simulink model "adaptiveFinal"  (R2014b)
settings: Solver=ode45  StartTime=0.0  StopTime=50.0  RelTol=1e-3
libraries: simulink x2
settings Model: Creator=highamj  LastModifiedBy=highamj

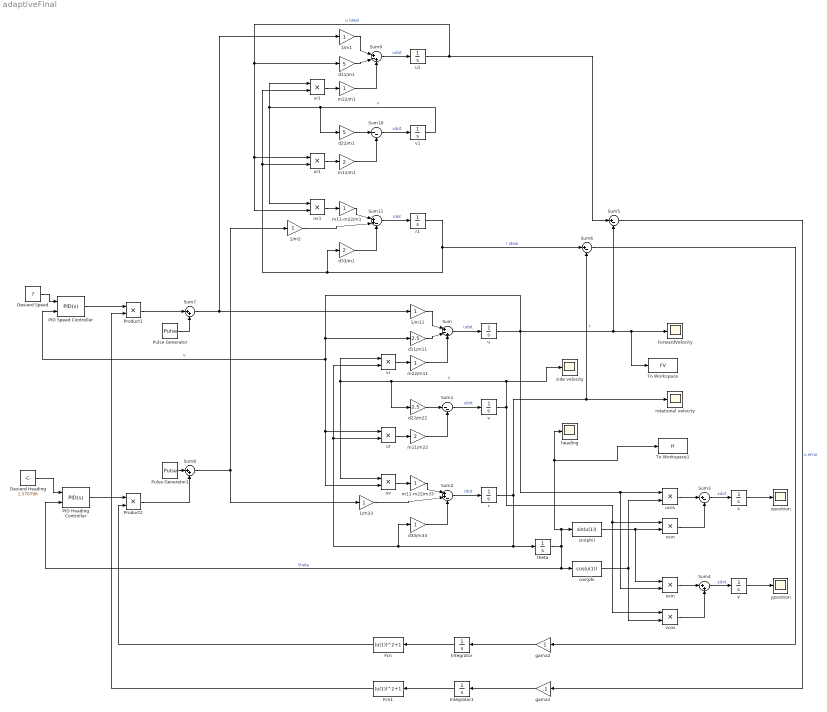
== system adaptiveFinal ==
  1/m{1..2,11,33} (4 alike) : Gain
  Desierd Heading : Constant  Value=1.570796
  Desierd Speed : Constant  Value=7
  Fcn : Fcn  Expr=(u(1))^2+1
  Fcn1 : Fcn  Expr=(u(1))^2+1
  ForwardVelocity : Scope
      settings: YMin=-2.92e+11  YMax=-2.86e+11  SaveName=ScopeData3
  Integrator : Integrator
  Integrator1 : Integrator
  PID Heading Controller : simulink/Continuous/PID Controller (2DOF)  Controller=PID  TimeDomain=Continuous-time  SampleTime=-1  IntegratorMethod=Forward Euler  FilterMethod=Forward Euler  Form=Parallel  P=5.96375779922345  I=0.127939709833734  D=1.41156755886535  N=5.23154506794489  b=1  c=1  InitialConditionSource=internal  InitialConditionForIntegrator=0  InitialConditionForFilter=0  ExternalReset=none  LimitOutput=off  UpperSaturationLimit=inf  LowerSaturationLimit=-inf  LinearizeAsGain=on  AntiWindupMode=none  Kb=1  TrackingMode=off  Kt=1  PParamMin=[]  PParamMax=[]  IParamMin=[]  IParamMax=[]  DParamMin=[]  DParamMax=[]  NParamMin=[]  NParamMax=[]  bParamMin=[]  bParamMax=[]  cParamMin=[]  cParamMax=[]  KbParamMin=[]  KbParamMax=[]  KtParamMin=[]  KtParamMax=[]  POutMin=[]  POutMax=[]  IOutMin=[]  IOutMax=[]  DOutMin=[]  DOutMax=[]  NOutMin=[]  NOutMax=[]  bOutMin=[]  bOutMax=[]  cOutMin=[]  cOutMax=[]  KbOutMin=[]  KbOutMax=[]  KtOutMin=[]  KtOutMax=[]  IntegratorOutMin=[]  IntegratorOutMax=[]  FilterOutMin=[]  FilterOutMax=[]  SumOutMin=[]  SumOutMax=[]  Sum1OutMin=[]  Sum1OutMax=[]  Sum2OutMin=[]  Sum2OutMax=[]  Sum3OutMin=[]  Sum3OutMax=[]  SumI1OutMin=[]  SumI1OutMax=[]  SumI2OutMin=[]  SumI2OutMax=[]  SumI3OutMin=[]  SumI3OutMax=[]  SumDOutMin=[]  SumDOutMax=[]  SaturationOutMin=[]  SaturationOutMax=[]  IntegratorContinuousStateAttributes=''  IntegratorStateMustResolveToSignalObject=off  IntegratorRTWStateStorageClass=Auto  FilterContinuousStateAttributes=''  FilterStateMustResolveToSignalObject=off  FilterRTWStateStorageClass=Auto  DifferentiatorICPrevScaledInput=0  DifferentiatorOutMin=[]  DifferentiatorOutMax=[]  UseFilter=on
  PID Speed Controller : simulink/Continuous/PID Controller (2DOF)  Controller=PID  TimeDomain=Continuous-time  SampleTime=-1  IntegratorMethod=Forward Euler  FilterMethod=Forward Euler  Form=Parallel  P=0  I=4.52260515354749  D=0  N=100  b=1  c=1  InitialConditionSource=internal  InitialConditionForIntegrator=0  InitialConditionForFilter=0  ExternalReset=none  LimitOutput=off  UpperSaturationLimit=inf  LowerSaturationLimit=-inf  LinearizeAsGain=on  AntiWindupMode=none  Kb=1  TrackingMode=off  Kt=1  PParamMin=[]  PParamMax=[]  IParamMin=[]  IParamMax=[]  DParamMin=[]  DParamMax=[]  NParamMin=[]  NParamMax=[]  bParamMin=[]  bParamMax=[]  cParamMin=[]  cParamMax=[]  KbParamMin=[]  KbParamMax=[]  KtParamMin=[]  KtParamMax=[]  POutMin=[]  POutMax=[]  IOutMin=[]  IOutMax=[]  DOutMin=[]  DOutMax=[]  NOutMin=[]  NOutMax=[]  bOutMin=[]  bOutMax=[]  cOutMin=[]  cOutMax=[]  KbOutMin=[]  KbOutMax=[]  KtOutMin=[]  KtOutMax=[]  IntegratorOutMin=[]  IntegratorOutMax=[]  FilterOutMin=[]  FilterOutMax=[]  SumOutMin=[]  SumOutMax=[]  Sum1OutMin=[]  Sum1OutMax=[]  Sum2OutMin=[]  Sum2OutMax=[]  Sum3OutMin=[]  Sum3OutMax=[]  SumI1OutMin=[]  SumI1OutMax=[]  SumI2OutMin=[]  SumI2OutMax=[]  SumI3OutMin=[]  SumI3OutMax=[]  SumDOutMin=[]  SumDOutMax=[]  SaturationOutMin=[]  SaturationOutMax=[]  IntegratorContinuousStateAttributes=''  IntegratorStateMustResolveToSignalObject=off  IntegratorRTWStateStorageClass=Auto  FilterContinuousStateAttributes=''  FilterStateMustResolveToSignalObject=off  FilterRTWStateStorageClass=Auto  DifferentiatorICPrevScaledInput=0  DifferentiatorOutMin=[]  DifferentiatorOutMax=[]  UseFilter=on
  Product1 : Product
  Product2 : Product
  Pulse Generator : DiscretePulseGenerator  PulseType=Time based  Amplitude=5  Period=5  PulseWidth=10
  Pulse Generator1 : DiscretePulseGenerator  PulseType=Time based  Amplitude=-1.570796  Period=25  PulseWidth=10
  Sum : Sum  Inputs=|+-+
  Sum1 : Sum  Inputs=|--
  Sum10 : Sum  Inputs=|--
  Sum11 : Sum  Inputs=|++-
  Sum2 : Sum  Inputs=|++-
  Sum3 : Sum  Inputs=|+-
  Sum4 : Sum  Inputs=|++
  Sum5 : Sum  Inputs=|+-
  Sum6 : Sum  Inputs=|+-
  Sum7 : Sum  Inputs=|++
  Sum8 : Sum  Inputs=|++
  Sum9 : Sum  Inputs=|+-+
  To Workspace : ToWorkspace  VariableName=FV  SaveFormat=Timeseries  SampleTime=-1
  To Workspace1 : ToWorkspace  VariableName=H  SaveFormat=Timeseries  SampleTime=-1
  cos(phi : Fcn  Expr=cos(u(1))
  d11/m1 : Gain  Gain=5
  d11/m11 : Gain  Gain=2.5
  d22/m1 : Gain  Gain=5
  d22/m22 : Gain  Gain=2.5
  d33/m1 : Gain  Gain=2
  d33/m33 : Gain
  gama1 : Gain  Gain=.1
  gama2 : Gain
  heading : Scope
      settings: YMin=-219000  YMax=-213000  SaveName=ScopeData2  SampleInput=on
  m11-m22/m1 : Gain
  m11-m22/m33 : Gain
  m11/m1 : Gain  Gain=2
  m11/m22 : Gain  Gain=2
  m22/m1 : Gain
  m22/m11 : Gain
  r : Integrator
  r1 : Integrator
  rotational velocity : Scope
      settings: SaveName=ScopeData4
  side velocity : Scope
      settings: SaveName=ScopeData5
  sin(phi) : Fcn  Expr=sin(u(1))
  theta : Integrator  InitialCondition=-0.785398
  u : Integrator
  u1 : Integrator
  ucos : Product
  ur : Product
  ur1 : Product
  usin : Product
  uv : Product
  uv1 : Product
  v : Integrator
  v1 : Integrator
  vcos : Product
  vr : Product
  vr1 : Product
  vsin : Product
  x : Integrator
  xposition : Scope
  y : Integrator
  yposition : Scope
  wires:
  vr/1 -> m22/m11/1
  v/1 -> vsin/1, vcos/1, side velocity/1, d22/m22/1, vr/1, uv/1  "v"
  r/1 -> vr/2, ur/2, d33/m33/1, theta/1, rotational velocity/1, Sum6/2  "r"
  Sum/1 -> u/1  "udot"
  Sum1/1 -> v/1  "vdot"
  Sum2/1 -> r/1  "rdot"
  m22/m11/1 -> Sum/3
  u/1 -> PID Speed Controller/2, uv/2, ur/1, d11/m11/1, Sum5/2, To Workspace/1, ForwardVelocity/1, ucos/1, usin/2  "u"
  d11/m11/1 -> Sum/2
  1/m11/1 -> Sum/1
  ur/1 -> m11/m22/1
  m11/m22/1 -> Sum1/2
  d22/m22/1 -> Sum1/1
  d33/m33/1 -> Sum2/3
  m11-m22/m33/1 -> Sum2/1
  uv/1 -> m11-m22/m33/1
  theta/1 -> To Workspace1/1, heading/1, sin(phi)/1, cos(phi/1, PID Heading Controller/2  "theta"
  Sum4/1 -> y/1  "ydot"
  Sum3/1 -> x/1  "xdot"
  sin(phi)/1 -> vsin/2, usin/1
  cos(phi/1 -> vcos/2, ucos/2
  ucos/1 -> Sum3/1
  vsin/1 -> Sum3/2
  usin/1 -> Sum4/1
  vcos/1 -> Sum4/2
  x/1 -> xposition/1
  y/1 -> yposition/1
  1/m33/1 -> Sum2/2
  u1/1 -> Sum5/1, uv1/2, ur1/1, d11/m1/1  "u ideal"
  r1/1 -> Sum6/1, vr1/2, ur1/2, d33/m1/1  "r ideal"
  Sum5/1 -> gama1/1  "u error"
  Fcn1/1 -> Product1/2
  Fcn/1 -> Product2/2
  Sum6/1 -> gama2/1
  vr1/1 -> m22/m1/1
  v1/1 -> d22/m1/1, vr1/1, uv1/1  "v"
  Sum9/1 -> u1/1  "udot"
  Sum10/1 -> v1/1  "vdot"
  Sum11/1 -> r1/1  "rdot"
  m22/m1/1 -> Sum9/3
  d11/m1/1 -> Sum9/2
  1/m1/1 -> Sum9/1
  ur1/1 -> m11/m1/1
  m11/m1/1 -> Sum10/2
  d22/m1/1 -> Sum10/1
  d33/m1/1 -> Sum11/3
  m11-m22/m1/1 -> Sum11/1
  uv1/1 -> m11-m22/m1/1
  1/m2/1 -> Sum11/2
  Desierd Speed/1 -> PID Speed Controller/1
  PID Speed Controller/1 -> Product1/1
  Desierd Heading/1 -> PID Heading Controller/1
  PID Heading Controller/1 -> Product2/1
  Pulse Generator/1 -> Sum7/2
  Product1/1 -> Sum7/1
  Sum7/1 -> 1/m1/1, 1/m11/1
  Pulse Generator1/1 -> Sum8/1
  Product2/1 -> Sum8/2
  Sum8/1 -> 1/m33/1, 1/m2/1
  gama2/1 -> Integrator/1
  Integrator/1 -> Fcn/1
  gama1/1 -> Integrator1/1
  Integrator1/1 -> Fcn1/1
